simulink model "metoda_kumpf"  (R2018a)
settings: Solver=VariableStepAuto  StartTime=0.0  StopTime=10.0  RelTol=1e-3
values from neighbouring files (symbols this model uses):
  K = 2    [ob_1.m]    (also in ob_2.m; ob_3.m)
  T_1 = 1    [ob_1.m]    (also in ob_2.m; ob_3.m)
  T_1_a = 0    [ob_1.m]    (also in ob_2.m; ob_3.m)
  T_1_b = T_1/10    (= 0.1)    [ob_1.m]    (also in ob_2.m; ob_3.m)
  T_1_c = T_1/2    (= 0.5)    [ob_1.m]    (also in ob_2.m; ob_3.m)
  T_1_d = T_1*1.05    (= 1.05)    [ob_1.m]    (also in ob_2.m; ob_3.m)
  T_a = 1.3    [ob_3.m]
  T_b = 1.4    [ob_3.m]
  T_c = 1.8    [ob_3.m]
  T_d = 1    [ob_1.m]    (also in ob_2.m; ob_3.m = 2.5)
settings Model: Creator=johnb  LastModifiedBy=johnb

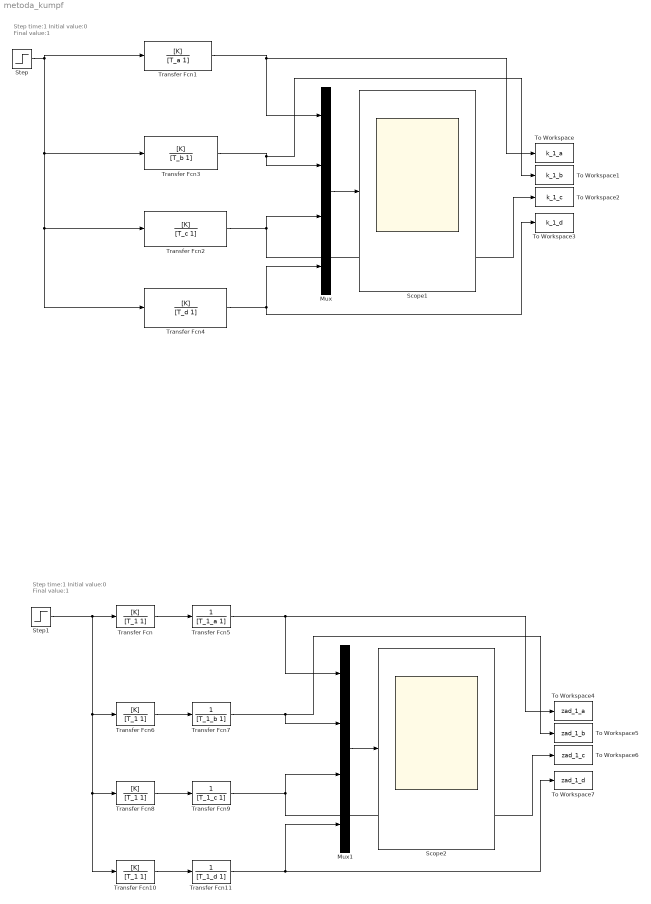
== system metoda_kumpf ==
  note: Step time:1
      | Initial value:0
      | Final value:1
  note: Step time:1
      | Initial value:0
      | Final value:1
  Mux : Mux
  Mux1 : Mux
  Scope1 : Scope
  Scope2 : Scope
  Step : Step  SampleTime=0
  Step1 : Step  SampleTime=0
  To Workspace : ToWorkspace  VariableName=k_1_a  SaveFormat=Timeseries  SampleTime=-1
  To Workspace1 : ToWorkspace  VariableName=k_1_b  SaveFormat=Timeseries  SampleTime=-1
  To Workspace2 : ToWorkspace  VariableName=k_1_c  SaveFormat=Timeseries  SampleTime=-1
  To Workspace3 : ToWorkspace  VariableName=k_1_d  SaveFormat=Timeseries  SampleTime=-1
  To Workspace4 : ToWorkspace  VariableName=zad_1_a  SaveFormat=Timeseries  SampleTime=-1
  To Workspace5 : ToWorkspace  VariableName=zad_1_b  SaveFormat=Timeseries  SampleTime=-1
  To Workspace6 : ToWorkspace  VariableName=zad_1_c  SaveFormat=Timeseries  SampleTime=-1
  To Workspace7 : ToWorkspace  VariableName=zad_1_d  SaveFormat=Timeseries  SampleTime=-1
  Transfer Fcn{,6,8,10} (4 alike) : TransferFcn  Numerator=[K]  Denominator=[T_1 1]
  Transfer Fcn1 : TransferFcn  Numerator=[K]  Denominator=[T_a 1]
  Transfer Fcn11 : TransferFcn  Denominator=[T_1_d 1]
  Transfer Fcn2 : TransferFcn  Numerator=[K]  Denominator=[T_c 1]
  Transfer Fcn3 : TransferFcn  Numerator=[K]  Denominator=[T_b 1]
  Transfer Fcn4 : TransferFcn  Numerator=[K]  Denominator=[T_d 1]
  Transfer Fcn5 : TransferFcn  Denominator=[T_1_a 1]
  Transfer Fcn7 : TransferFcn  Denominator=[T_1_b 1]
  Transfer Fcn9 : TransferFcn  Denominator=[T_1_c 1]
  wires:
  Transfer Fcn3/1 -> To Workspace1/1, Mux/2
  Transfer Fcn4/1 -> To Workspace3/1, Mux/4
  Transfer Fcn1/1 -> To Workspace/1, Mux/1
  Step/1 -> Transfer Fcn1/1, Transfer Fcn4/1, Transfer Fcn2/1, Transfer Fcn3/1
  Mux/1 -> Scope1/1
  Transfer Fcn2/1 -> To Workspace2/1, Mux/3
  Transfer Fcn/1 -> Transfer Fcn5/1
  Transfer Fcn9/1 -> To Workspace6/1, Mux1/3
  Transfer Fcn6/1 -> Transfer Fcn7/1
  Transfer Fcn11/1 -> To Workspace7/1, Mux1/4
  Transfer Fcn10/1 -> Transfer Fcn11/1
  Step1/1 -> Transfer Fcn10/1, Transfer Fcn8/1, Transfer Fcn6/1, Transfer Fcn/1
  Transfer Fcn7/1 -> To Workspace5/1, Mux1/2
  Transfer Fcn5/1 -> To Workspace4/1, Mux1/1
  Transfer Fcn8/1 -> Transfer Fcn9/1
  Mux1/1 -> Scope2/1
